simulink model "simucheck"  (R2021b)
settings: Solver=VariableStepAuto  StartTime=0.0  StopTime=10  RelTol=1e-3
undefined symbols (not defined in the file or in its folder): den, DiscIntNeverNeededParam, Gden, Gnum, num, q6, q7
libraries: eeLuenbergerObserver x1
settings Model: Creator=wvand  LastModifiedBy=wvand

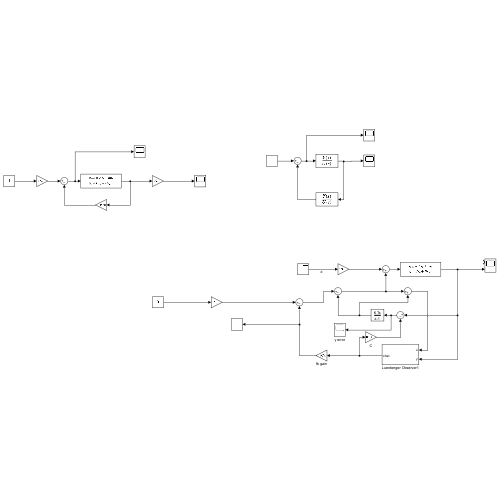
[thumbnail: Simulink's stored preview of the top-level diagram]
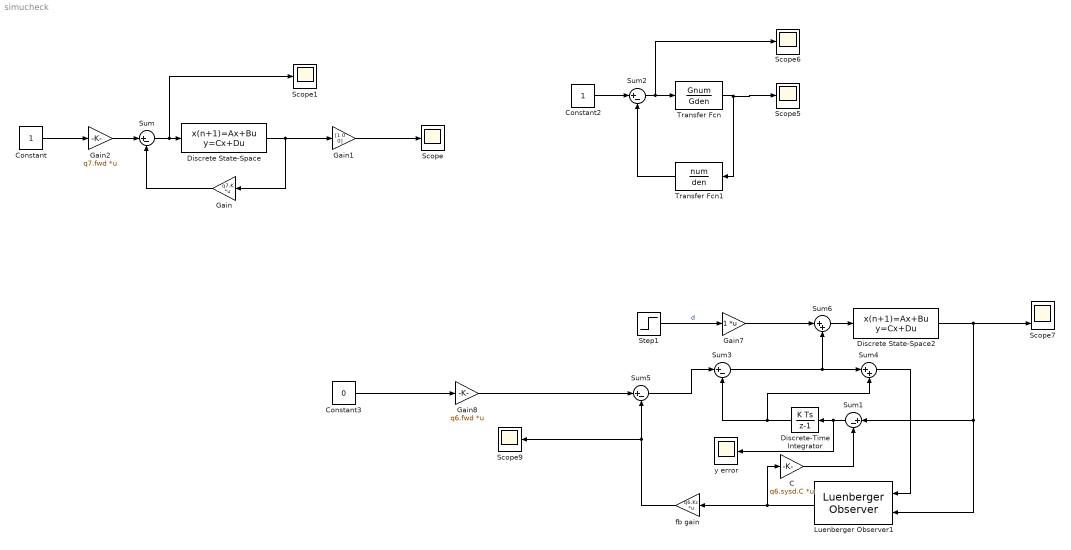
== system simucheck ==
  C : Gain  Gain=q6.sysd.C  Multiplication=Matrix(K*u)
  Constant : Constant  SampleTime=-1
  Constant2 : Constant  SampleTime=-1
  Constant3 : Constant  Value=0  SampleTime=-1
  Discrete State-Space : DiscreteStateSpace  A=q7.sysd.A  B=q7.sysd.B  C=eye(3)  D=zeros(3,1)  SampleTime=0.008
  Discrete State-Space2 : DiscreteStateSpace  A=q6.sysd.A  B=q6.sysd.B  C=q6.sysd.C  D=zeros(1,1)  SampleTime=q6.h
  Discrete-Time Integrator : DiscreteIntegrator  gainval=1000  SampleTime=-1  ICPrevOutput=DiscIntNeverNeededParam  ICPrevScaledInput=DiscIntNeverNeededParam
  Gain : Gain  Gain=q7.K  Multiplication=Matrix(K*u)
  Gain1 : Gain  Gain=[1 0 0]
  Gain2 : Gain  Gain=q7.fwd  Multiplication=Matrix(K*u)
  Gain7 : Gain  Multiplication=Matrix(K*u)
  Gain8 : Gain  Gain=q6.fwd  Multiplication=Matrix(K*u)
  Luenberger Observer1 : eeLuenbergerObserver/Luenberger Observer  StateSpaceType=Discrete-time  Ad=q6.sysd.A  Bd=q6.sysd.B  Cd=q6.sysd.C  Dd=q6.sysd.D  A=1  B=1  C=1  D=1  ObserverDesign=Observer gain  Ld=q6.Lo  DesiredEigenvalues=0  x0=[0 0 0]'  Tsd=0.1  Ts=-1
      settings: SourceProductBaseCode=PS
  Scope{,1,5..6,9} (5 alike) : Scope
  Scope7 : Scope  NumInputPorts=2
  Step1 : Step  SampleTime=0
  Sum{,1..3,5} (5 alike) : Sum  Inputs=|+-
  Sum4 : Sum  Inputs=|++
  Sum6 : Sum  Inputs=|++
  Transfer Fcn : TransferFcn  Numerator=Gnum  Denominator=Gden
  Transfer Fcn1 : TransferFcn  Numerator=num  Denominator=den
  fb gain : Gain  Gain=q6.Kc  Multiplication=Matrix(K*u)
  y error : Scope
  wires:
  Discrete State-Space/1 -> Gain/1, Gain1/1
  Gain2/1 -> Sum/1
  Sum/1 -> Scope1/1, Discrete State-Space/1
  Gain/1 -> Sum/2
  Constant/1 -> Gain2/1
  Gain1/1 -> Scope/1
  Constant2/1 -> Sum2/1
  Transfer Fcn/1 -> Scope5/1, Transfer Fcn1/1
  Sum2/1 -> Scope6/1, Transfer Fcn/1
  Transfer Fcn1/1 -> Sum2/2
  Gain8/1 -> Sum5/1
  Gain7/1 -> Sum6/1
  Step1/1 -> Gain7/1  "d"
  fb gain/1 -> Scope9/1, Sum5/2
  Constant3/1 -> Gain8/1
  Sum6/1 -> Discrete State-Space2/1
  Luenberger Observer1/1 -> fb gain/1, C/1
  Discrete State-Space2/1 -> Sum1/1, Luenberger Observer1/2, Scope7/2
  C/1 -> Sum1/2
  Sum1/1 -> y error/1, Discrete-Time Integrator/1
  Sum5/1 -> Sum3/1
  Sum3/1 -> Sum4/1, Sum6/2
  Discrete-Time Integrator/1 -> Sum4/2, Sum3/2
  Sum4/1 -> Luenberger Observer1/1
